simulink model "task_2_simm"  (R2023a)
settings: Solver=VariableStepAuto  StartTime=0.0  StopTime=5  MaxStep=1e-4  RelTol=1e-5
undefined symbols (not defined in the file): A, C, L, x0, xh0
settings Model: Creator=user  LastModifiedBy=user

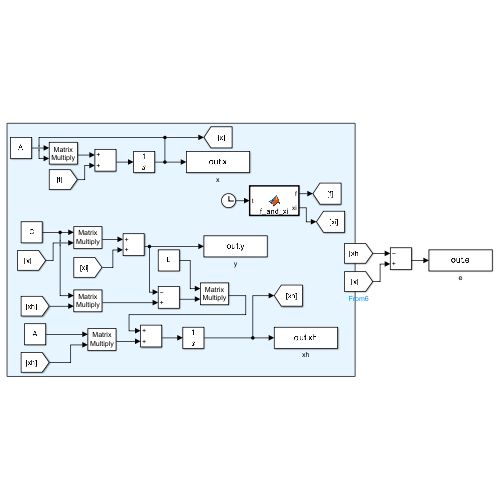
[thumbnail: Simulink's stored preview of the top-level diagram]
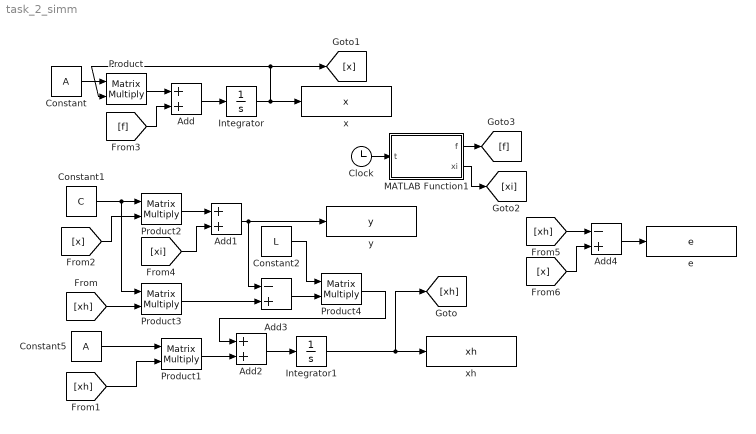
== system task_2_simm ==
  Add : Sum
  Add1 : Sum
  Add2 : Sum
  Add3 : Sum  Inputs=-+
  Add4 : Sum  Inputs=-+
  Clock : Clock
  Constant : Constant  Value=A  VectorParams1D=off
  Constant1 : Constant  Value=C  VectorParams1D=off
  Constant2 : Constant  Value=L  VectorParams1D=off
  Constant5 : Constant  Value=A  VectorParams1D=off
  Integrator : Integrator  InitialCondition=x0
  Integrator1 : Integrator  InitialCondition=xh0
  MATLAB Function1 : MATLAB Function  TreatAsAtomicUnit=on
  Product{,1..4} (5 alike) : Product  Multiplication=Matrix(*)
  e : ToWorkspace  VariableName=e  SaveFormat=Timeseries  SampleTime=-1
  x : ToWorkspace  VariableName=x  SaveFormat=Timeseries  SampleTime=-1
  xh : ToWorkspace  VariableName=xh  SaveFormat=Timeseries  SampleTime=-1
  y : ToWorkspace  VariableName=y  SaveFormat=Timeseries  SampleTime=-1
  wires:
  Constant/1 -> Product/1
  Product/1 -> Add/1
  [f] -> Add/2
  Add/1 -> Integrator/1
  Integrator/1 -> x/1, [x], Product/2
  Constant1/1 -> Product3/1, Product2/1
  Product2/1 -> Add1/1
  [xi] -> Add1/2
  Add1/1 -> y/1, Add3/1
  Integrator1/1 -> xh/1, [xh]
  Constant5/1 -> Product1/1
  Product1/1 -> Add2/2
  Product3/1 -> Add3/2
  Add3/1 -> Product4/2
  Constant2/1 -> Product4/1
  Product4/1 -> Add2/1
  Add2/1 -> Integrator1/1
  [xh] -> Product1/2
  [xh] -> Product3/2
  [x] -> Product2/2
  Clock/1 -> MATLAB Function1/1(t)
  MATLAB Function1/1(f) -> [f]
  MATLAB Function1/2(xi) -> [xi]
  Add4/1 -> e/1
  [xh] -> Add4/1
  [x] -> Add4/2

== matlab function task_2_simm/MATLAB Function1 ==
  data: t input; f output; xi output
function [f, xi] = f_and_xi(t)
    f = [0.5*sin(2*pi*0.1*t);
         0.3*cos(2*pi*0.2*t);
         0.4*sin(2*pi*0.15*t);
         0.2*cos(2*pi*0.05*t)];
    
    xi = 0.1*sin(2*pi*0.3*t) + 0.05*cos(2*pi*0.25*t);
end
